simulink model "stepRecovery"  (Simulink 8.7)
settings: Solver=FixedStepDiscrete  StartTime=0.0  StopTime="CONFIG.SIMULATION_TIME "  FixedStep=CONFIG.Ts  RelTol=1e-3
InitFcn:
  | cd(fileparts(which(bdroot)));
  | initStepRecovery;
values from neighbouring files (symbols this model uses):
  baseToWorldRotationPort = '/matlabTorqueBalancing/floatingBaseRotationMatrix:i'    [esperimento_fake2.mat]    (also in initStepRecovery.m = ['/' WBT_modelName '/floatingBaseRotationMatrix:i']; initTorqueBalancing.m = ['/' WBT_modelName '/floatingBaseRotationMatrix:i']; secondo_risultato.mat)
  bVectorConstraints = [0 0 0 0 0 0 0 0 0 0 0 0 ... (19 elements, 19x1)]    [esperimento_fake2.mat]    (also in secondo_risultato.mat)
  CONFIG =     [esperimento_fake2.mat]    (also in secondo_risultato.mat)
  ConstraintsMatrix = [3.73205080757 1 0.267949192431 -0.267949192431 -1 -3.73205080757 -3.73205080757 -1 -0.267949192431 0.267949192431 1 3.73205080757 ... (114 elements, 19x6)]    [esperimento_fake2.mat]    (also in secondo_risultato.mat)
  gain =     [esperimento_fake2.mat]    (also in secondo_risultato.mat)
  references =     [esperimento_fake2.mat]    (also in secondo_risultato.mat)
  reg =     [esperimento_fake2.mat]    (also in secondo_risultato.mat)
  ROBOT_DOF = 23    [esperimento_fake2.mat]    (also in secondo_risultato.mat)
  ROBOT_DOF_FOR_SIMULINK = [1 0 0 0 0 0 0 0 0 0 0 0 ... (529 elements, 23x23)]    [esperimento_fake2.mat]    (also in secondo_risultato.mat)
  sat =     [esperimento_fake2.mat]    (also in secondo_risultato.mat)
  SM =     [esperimento_fake2.mat]    (also in secondo_risultato.mat)
  sm =     [esperimento_fake2.mat]    (also in secondo_risultato.mat)
  WBT_modelName = 'matlabTorqueBalancing'    [esperimento_fake2.mat]    (also in initStepRecovery.m; initTorqueBalancing.m; secondo_risultato.mat)
  WBT_robotName = ''    [esperimento_fake2.mat]    (also in secondo_risultato.mat)
undefined symbols (not defined in the file or in its folder): DiscIntNeverNeededParam
libraries: WBToolboxLibrary x171, simulink x16, simulink_extras x4
(part 5 of 5)

== matlab function DesValues/State Machine Step Recovery/visualise inertial/Visualize hom transf6/MATLAB Function ==
  data: R input double; rollPitchYaw output double
function rollPitchYaw = buildHomogenousTranformation(R)
%#codegen

rollPitchYaw = rollPitchYawFromRotation(R);

rollPitchYaw = rollPitchYaw*180/pi;

== matlab function DesValues/State Machine Step Recovery/visualise inertial/w_H_root_link1/fromImuToHomogeousTransformFCN ==
  data: imu_H_link input double; imu_H_link_0 input double; link_H_root input double; inertial_0 input double; inertial input double; neck input double; w_H_root output double; CONFIG parameter double
function w_H_root = fromBaseToWorldWithImuFCN(imu_H_link,imu_H_link_0,link_H_root,inertial_0,inertial,neck,CONFIG)
%#codegen
w_H_root = fromBaseToWorldWithImu(imu_H_link,imu_H_link_0,link_H_root,inertial_0,inertial,neck,CONFIG);

== matlab function DesValues/State Machine Step Recovery/visualise inertial/w_H_root_link4/fromImuToHomogeousTransformFCN ==
  data: imu_H_link input double; imu_H_link_0 input double; link_H_root input double; inertial_0 input double; inertial input double; neck input double; w_H_root output double; CONFIG parameter double
function w_H_root = fromBaseToWorldWithImuFCN(imu_H_link,imu_H_link_0,link_H_root,inertial_0,inertial,neck,CONFIG)
%#codegen
w_H_root = fromBaseToWorldWithImu(imu_H_link,imu_H_link_0,link_H_root,inertial_0,inertial,neck,CONFIG);

== matlab function DesValues/State Machine Step Recovery/w_H_root_link1/fromImuToHomogeousTransformFCN ==
  data: imu_H_link input double; imu_H_link_0 input double; link_H_root input double; inertial_0 input double; inertial input double; neck input double; w_H_root output double; CONFIG parameter double
function w_H_root = fromBaseToWorldWithImuFCN(imu_H_link,imu_H_link_0,link_H_root,inertial_0,inertial,neck,CONFIG)
%#codegen
w_H_root = fromBaseToWorldWithImu(imu_H_link,imu_H_link_0,link_H_root,inertial_0,inertial,neck,CONFIG);

== matlab function DesValues/State Machine Step Recovery/w_H_root_link4/fromImuToHomogeousTransformFCN ==
  data: imu_H_link input double; imu_H_link_0 input double; link_H_root input double; inertial_0 input double; inertial input double; neck input double; w_H_root output double; CONFIG parameter double
function w_H_root = fromBaseToWorldWithImuFCN(imu_H_link,imu_H_link_0,link_H_root,inertial_0,inertial,neck,CONFIG)
%#codegen
w_H_root = fromBaseToWorldWithImu(imu_H_link,imu_H_link_0,link_H_root,inertial_0,inertial,neck,CONFIG);

== matlab function DesValues/State Machine Step Recovery/Step Recovery reference generator/Step Recovery Techniques /FPE module/MATLAB Function ==
  data: base_origin input double; Mbb input double; Mbb_COM output double; COMx input double
function Mbb_COM  = COM_inertia_matrix_sim(base_origin, Mbb, COMx)
Mbb_COM = COM_inertia_matrix(Mbb, base_origin, COMx);

== matlab function DesValues/State Machine Step Recovery/Step Recovery reference generator/Step Recovery Techniques /Capture Point Computer/Capture Point-alternative/MATLAB Function ==
  data: omega input double; r_CP output double; r_ic input double; r_CxP input double; robot_step_time input double; STEP input double; delta_t input double
function r_CP = capture_point(omega, r_ic, r_CxP, robot_step_time, STEP, delta_t)
 persistent elapsed_time;
 
 if isempty(elapsed_time)
     elapsed_time = 0;
 end
 
 if (STEP == 0)
     r_CP = r_ic;
     elapsed_time = 0;
 
 else  r_CP = (r_ic - r_CxP)*exp(omega * (robot_step_time-elapsed_time)) + r_CxP;
       if (elapsed_time < (robot_step_time-delta_t))
           elapsed_time = elapsed_time + delta_t;
       end
 end
end

== matlab function DesValues/State Machine Step Recovery/Step Recovery reference generator/Step Recovery Techniques /FPE module/MATLAB Function2 ==
  data: m input double; COMx input double; COM_vel input double; J_COM input double; g input double; theta_bar output double; foot input double; x output double
function [theta_bar, x] = fpe_sim(m, COMx, COM_vel, J_COM, g, foot)
 [theta_bar, x] = fpe_computation(m, COMx, COM_vel, J_COM, g, foot);

== matlab function DesValues/State Machine Step Recovery/Step Recovery reference generator/Step Recovery Techniques /FPE module/Out of left foot_CH/Inverse ==
  data: w_H_a input double; a_H_w output double
function a_H_w = inverse(w_H_a)

R = w_H_a(1:3,1:3);
p = w_H_a(1:3,4);

a_H_w = [R',        -R'*p;
        zeros(1,3),     1];

== matlab function DesValues/State Machine Step Recovery/Step Recovery reference generator/Step Recovery Techniques /Capture Point Computer/Out of left foot_CH/Inverse ==
  data: w_H_a input double; a_H_w output double
function a_H_w = inverse(w_H_a)

R = w_H_a(1:3,1:3);
p = w_H_a(1:3,4);

a_H_w = [R',        -R'*p;
        zeros(1,3),     1];

== matlab function DesValues/State Machine Step Recovery/Step Recovery reference generator/Step Recovery Techniques /FPE module/Out of left foot_CH/MATLAB Function ==
  data: x input double; OUT output double; w_H_lsole input double; w_H_rsole input double; foot_size input double
function OUT = in_convex_hull(x,w_H_lsole, w_H_rsole, foot_size)
OUT = in_convex_hull(x,w_H_lsole, w_H_rsole, foot_size);

== matlab function DesValues/State Machine Step Recovery/Step Recovery reference generator/Step Recovery Techniques /Capture Point Computer/Capture Point/MATLAB Function1 ==
  data: omega input double; r input double; r_eq output double; delta_t input double; OUT input double
function r_eq = equivalent_r (omega, r, delta_t, OUT)
r_eq = equivalent_r (r, delta_t, omega, OUT);

== matlab function DesValues/State Machine Step Recovery/Step Recovery reference generator/Step Recovery Techniques /Capture Point Computer/Capture Point/MATLAB Function ==
  data: omega input double; r_CP output double; r_ic input double; r_CxP input double; robot_step_time input double; STEP input double
function r_CP = capture_point(omega, r_ic, r_CxP, robot_step_time, STEP)
r_CP = capture_point(STEP, r_ic, r_CxP, omega, robot_step_time);

== matlab function DesValues/State Machine Step Recovery/Step Recovery reference generator/Inverse Kinematics/MATLAB Function ==
  data: des_pos input double; w_H_f output double; rot_x input double; rot_y input double; rot_z input double
function w_H_f = desired_transformation (des_pos,rot_x, rot_y, rot_z)

des_pos = reshape(des_pos,3,1);
R=eul2rotm([rot_z,rot_y,rot_x]);

w_H_f = [R    ,des_pos; 
         zeros(1,3),1];

== matlab function DesValues/State Machine Step Recovery/Step Recovery reference generator/Step Recovery Techniques /ankle, CoP, Cmp (LEFT FOOT)/CMP computer/MATLAB Function ==
  data: R input double; s_A_b output double; p input double
function s_A_b = adjoint (R,p)
s_A_b = adjoint (R,p);

== matlab function DesValues/State Machine Step Recovery/Step Recovery reference generator/Step Recovery Techniques /Capture Point Computer/Capture Point/Versor ==
  data: r_CxP input double; omega input double; r_ic input double; direction output double
function direction = CP_direction(r_CxP, omega, r_ic)

r_ic_dot = omega*(r_ic - r_CxP);

if(norm(r_ic_dot,2) > 0)
    direction = r_ic_dot/norm(r_ic_dot,2);
else direction = zeros(length(r_ic_dot),1);
end

end

== matlab function DesValues/State Machine Step Recovery/Step Recovery reference generator/Step Recovery Techniques /FPE module/Out of left foot_CH/Out of left foot  ==
  data: x input double; OUT output double; support input double; shadow input double; OUT_real output double
function [OUT, OUT_real] = exit_support_square_shadowed(x, support,shadow)
%computes whether x is outside the support polygon defined in supportp. x
%should be a two dimensional vector, while supportp a 2x2 matrix, where
%the first coloumn is the lower edge, while the first row corresponds to
%the first dimension of x. Notice that this check is done only if x is
%inside the shadowed region.
[OUT, OUT_real] = exit_support_square_shadowed(x, support, shadow);

== matlab function DesValues/State Machine Step Recovery/Step Recovery reference generator/Selector and Saturation/MATLAB Function ==
  data: x input double; x_sat output double; max_d input double; SAT output double; min_d input double
function [x_sat, SAT]=step_saturation(x,max_d,min_d)
[x_sat, SAT]=step_saturation(x,max_d,min_d);

== matlab function DesValues/State Machine Step Recovery/Step Recovery reference generator/Step Recovery Techniques /Capture Point Computer/Out of left foot_CH/MATLAB Function ==
  data: x input double; OUT output double; w_H_lsole input double; w_H_rsole input double; foot_size input double
function OUT = in_convex_hull(x,w_H_lsole, w_H_rsole, foot_size)
OUT = in_convex_hull(x,w_H_lsole, w_H_rsole, foot_size);

== matlab function DesValues/State Machine Step Recovery/Step Recovery reference generator/Step Recovery Techniques /FPE module/MATLAB Function3 ==
  data: theta_bar input double; fpe output double; COMx input double; x input double; offset input double; fpe_offset output double
function [fpe, fpe_offset] = fpe_pos(theta_bar, COMx, x, offset)
h = COMx(3);
fpe = h*tan(theta_bar)*x + [COMx(1);COMx(2);0];
fpe_offset = h*tan(theta_bar+offset)*x + [COMx(1);COMx(2);0];

== matlab function DesValues/State Machine Step Recovery/Step Recovery reference generator/Step Recovery Techniques /Capture Point Computer/Out of left foot_CH/Out of left foot  ==
  data: x input double; OUT output double; support input double; shadow input double; OUT_real output double
function [OUT, OUT_real] = exit_support_square_shadowed(x, support,shadow)
%computes whether x is outside the support polygon defined in supportp. x
%should be a two dimensional vector, while supportp a 2x2 matrix, where
%the first coloumn is the lower edge, while the first row corresponds to
%the first dimension of x. Notice that this check is done only if x is
%inside the shadowed region.
[OUT, OUT_real] = exit_support_square_shadowed(x, support, shadow);

== matlab function DesValues/State Machine Step Recovery/Step Recovery reference generator/Inverse Kinematics/Inverse ==
  data: w_H_a input double; a_H_w output double
function a_H_w = inverse(w_H_a)

R = w_H_a(1:3,1:3);
p = w_H_a(1:3,4);

a_H_w = [R',        -R'*p;
        zeros(1,3),     1];

== matlab function DesValues/State Machine Step Recovery/Visualize hom transf5/MATLAB Function ==
  data: R input double; rollPitchYaw output double
function rollPitchYaw = buildHomogenousTranformation(R)
%#codegen

rollPitchYaw = rollPitchYawFromRotation(R);

rollPitchYaw = rollPitchYaw*180/pi;
